simulink model "rate_controller_model"  (R2016a)
settings: Solver=VariableStepAuto  StartTime=0.0  StopTime=10.0  RelTol=1e-3
settings Model: Creator=GusBus  LastModifiedBy=GusBus
settings DataIOCC: LimitDataPoints=on
settings DebuggingCC: AllowSymbolicDim=off
settings ModelReferenceCC: PropagateSignalLabelsOutOfModel=off
settings GRTTargetCC: GeneratePreprocessorConditionals=Use local settings

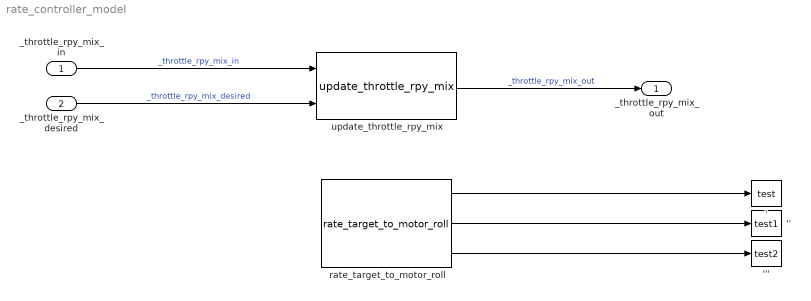
== system rate_controller_model ==
  _throttle_rpy_mix_in : Inport
  _throttle_rpy_mix_desired : Inport  Port=2
  ' : ToWorkspace  VariableName=test  SaveFormat=Timeseries  SampleTime=-1
  '' : ToWorkspace  VariableName=test1  SaveFormat=Timeseries  SampleTime=-1
  ''' : ToWorkspace  VariableName=test2  SaveFormat=Timeseries  SampleTime=-1
  rate_target_to_motor_roll : S-Function  FunctionName=rate_target_to_motor_roll  SFunctionDeploymentMode=off  EnableBusSupport=off
  update_throttle_rpy_mix : S-Function  FunctionName=update_throttle_rpy_mix  SFunctionDeploymentMode=off  EnableBusSupport=off
  _throttle_rpy_mix_out : Outport
  wires:
  _throttle_rpy_mix_in/1 -> update_throttle_rpy_mix/1  "_throttle_rpy_mix_in"
  rate_target_to_motor_roll/1 -> '/1
  rate_target_to_motor_roll/3 -> '''/1
  rate_target_to_motor_roll/2 -> ''/1
  update_throttle_rpy_mix/1 -> _throttle_rpy_mix_out/1  "_throttle_rpy_mix_out"
  _throttle_rpy_mix_desired/1 -> update_throttle_rpy_mix/2  "_throttle_rpy_mix_desired"
